simulink model "Franklin_ex_7_2_sim"  (R2024b)
settings: Solver=VariableStepAuto  StartTime=0.0  StopTime=150  RelTol=1e-3
values from neighbouring files (symbols this model uses):
  b = 60    [Franklin_ex_7_2.m]
  m = 1500    [Franklin_ex_7_2.m]
settings Model: Creator=Nico  LastModifiedBy=Nico

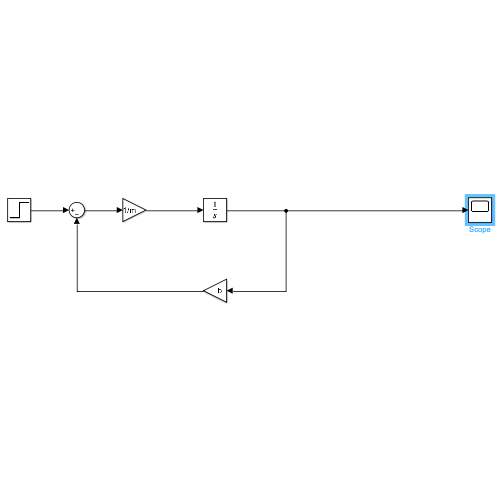
[thumbnail: Simulink's stored preview of the top-level diagram]
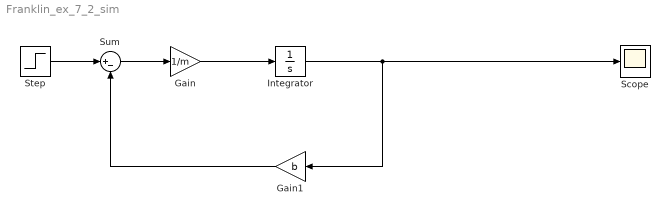
== system Franklin_ex_7_2_sim ==
  Gain : Gain  Gain=1/m
  Gain1 : Gain  Gain=b
  Integrator : Integrator
  Scope : Scope
  Step : Step  Time=0  After=750  SampleTime=0
  Sum : Sum  Inputs=|+-
  wires:
  Step/1 -> Sum/1
  Sum/1 -> Gain/1
  Gain/1 -> Integrator/1
  Integrator/1 -> Scope/1, Gain1/1
  Gain1/1 -> Sum/2
